simulink model "example_iec61850"  (Simulink 8.1)
settings: Solver=FixedStepDiscrete  SolverMode=SingleTasking  StartTime=0.0  StopTime=Inf  FixedStep=0.00025  RelTol=1e-3
PostLoadFcn:
  | Ts=0.02; Ns=4; txnb=0; rxnb=0;
InitFcn:
  | Ts=0.02; Ns=4; txnb=0; rxnb=0;
undefined symbols (not defined in the file): CD
libraries: opal_lib x6, simulink x6, rtio_iec61850 x4, rtlab x2
settings Model: Creator=CristinaO  LastModifiedBy=pkoralew  BufferReuse=off
settings DataIOCC: SaveOutput=off  SignalLogging=off  SaveTime=off
settings OptimizationCC: BlockReduction=off  OptimizeBlockIOStorage=off  BufferReuse=off  ExpressionFolding=off  LocalBlockOutputs=off  InitFltsAndDblsToZero=on
settings DebuggingCC: SaveWithParameterizedLinksMsg=none  StrictBusMsg=Warning
settings HardwareCC: TargetHWDeviceType=32-bit Generic
settings GRTTargetCC: TargetFcnLib=ansi_tfl_tmw.mat

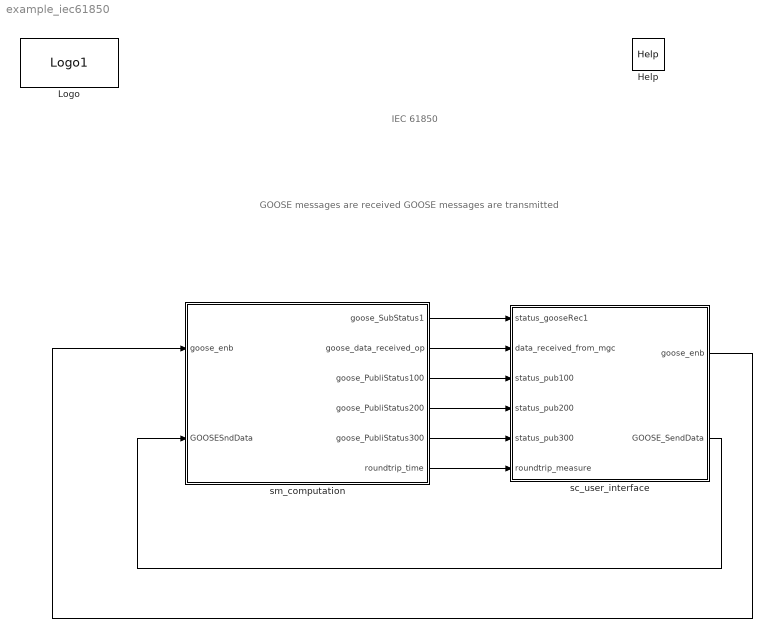
== system example_iec61850 ==
  note: GOOSE messages are received
      |
      | GOOSE messages are transmitted
  note: IEC 61850
  Help : opal_lib/Help  docfile=../help/help.html
  Logo : opal_lib/Logo1  vide=[]
  sc_user_interface : Subsystem
  sm_computation : Subsystem
  wires:
  sm_computation/1(goose_SubStatus1) -> sc_user_interface/1(status_gooseRec1)
  sm_computation/2(goose_data_received_op) -> sc_user_interface/2(data_received_from_mgc)
  sc_user_interface/1(goose_enb) -> sm_computation/1(goose_enb)
  sc_user_interface/2(GOOSE_SendData) -> sm_computation/2(GOOSESndData)
  sm_computation/3("goose_PubliStatus100 ") -> sc_user_interface/3(status_pub100)
  sm_computation/4(goose_PubliStatus200) -> sc_user_interface/4(status_pub200)
  sm_computation/5(goose_PubliStatus300) -> sc_user_interface/5(status_pub300)
  sm_computation/6(roundtrip_time) -> sc_user_interface/6(roundtrip_measure)

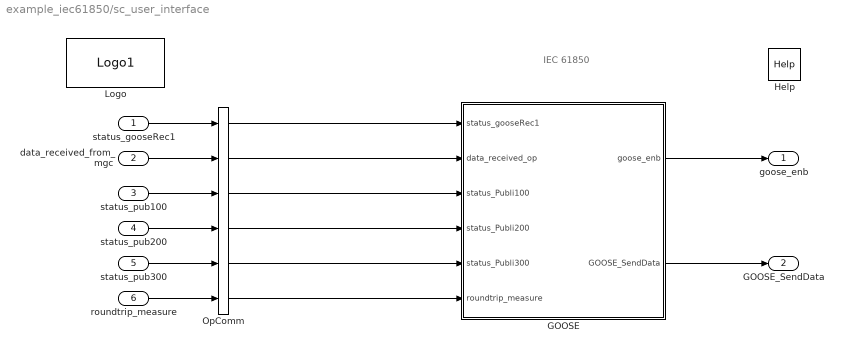
== system example_iec61850/sc_user_interface ==
  note: IEC 61850
  status_gooseRec1 : Inport
  data_received_from_mgc : Inport  Port=2
  status_pub100 : Inport  Port=3
  status_pub200 : Inport  Port=4
  status_pub300 : Inport  Port=5
  roundtrip_measure : Inport  Port=6
  GOOSE : Subsystem
  Help : opal_lib/Help  docfile=../help/help.html
  Logo : opal_lib/Logo1  vide=[]
  OpComm : rtlab/OpComm  nbport=6  groupe_acq=1  subsys_rate=0  st=0  Synchronization=off  Interpolation=off  Threshold=1.0  Missed_Data=off  Sim_Time=off  Samples=off  dynSigOut=off  from_console=0  warning_done=off  writeOpCommFile=off  Offset=off
  goose_enb : Outport
  GOOSE_SendData : Outport  Port=2
  wires:
  status_gooseRec1/1 -> OpComm/1
  data_received_from_mgc/1 -> OpComm/2
  GOOSE/1(goose_enb) -> goose_enb/1
  GOOSE/2(GOOSE_SendData) -> GOOSE_SendData/1
  OpComm/1 -> GOOSE/1(status_gooseRec1)
  OpComm/2 -> GOOSE/2(data_received_op)
  status_pub300/1 -> OpComm/5
  status_pub100/1 -> OpComm/3
  status_pub200/1 -> OpComm/4
  OpComm/5 -> GOOSE/5(status_Publi300)
  OpComm/3 -> GOOSE/3(status_Publi100)
  OpComm/4 -> GOOSE/4(status_Publi200)
  roundtrip_measure/1 -> OpComm/6
  OpComm/6 -> GOOSE/6(roundtrip_measure)

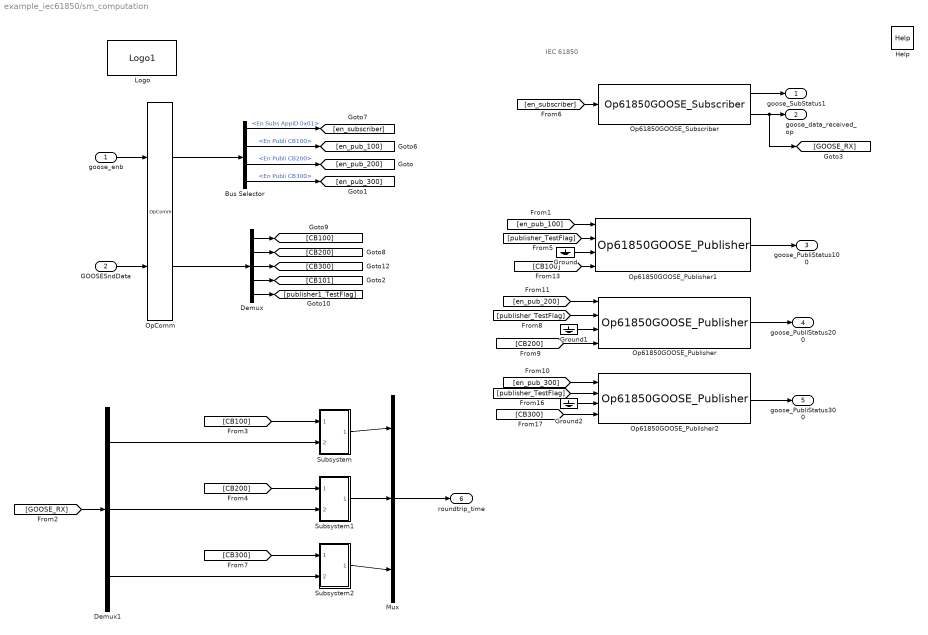
== system example_iec61850/sm_computation ==
  note: IEC 61850
  goose_enb : Inport
  GOOSESndData : Inport  Port=2
  Bus Selector : BusSelector  OutputSignals=En Subs AppID 0x01,En Publi CB100,En Publi CB200,En Publi CB300
  Demux : Demux  Outputs=5
  Demux1 : Demux  Outputs=3
  Ground : Ground
  Ground1 : Ground
  Ground2 : Ground
  Help : opal_lib/Help  docfile=../help/help.html
  Logo : opal_lib/Logo1  vide=[]
  Mux : Mux  Inputs=3
  Op61850GOOSE_Publisher : rtio_iec61850/Op61850GOOSE_Publisher  nic_name=eth1  ied_name=CB200  select_scl=off  scl_file=CB200.icd  scl_fullpath=.  goose_name=Goose_TRIP1  goose_msgid=0x0200  mac_address=01-0C-CD-01-28-50  vlan_prio=4  vlan_id=000  mintime=25  maxtime=250  gocbref=CB200LDevice1/LLN0$GO$CB_Goose_TRIP1  dataset=CB200LDevice1/LLN0$Goose_TRIP1  goID=Goose_TRIP1  confrev=1  externalClock=off
      settings: AttributesFormatString=%<Name>\nAppId = %<goose_msgid>
  Op61850GOOSE_Publisher1 : rtio_iec61850/Op61850GOOSE_Publisher  nic_name=eth1  ied_name=CB100  select_scl=off  scl_file=CB100.icd  scl_fullpath=.  goose_name=Goose_TRIP1  goose_msgid=0x0100  mac_address=01-0C-CD-01-28-50  vlan_prio=4  vlan_id=000  mintime=25  maxtime=250  gocbref=CB100LDevice1/LLN0$GO$CB_Goose_TRIP1  dataset=CB100LDevice1/LLN0$Goose_TRIP1  goID=Goose_TRIP1  confrev=1  externalClock=off
      settings: AttributesFormatString=%<Name>\nAppId = %<goose_msgid>
  Op61850GOOSE_Publisher2 : rtio_iec61850/Op61850GOOSE_Publisher  nic_name=eth1  ied_name=CB300  select_scl=off  scl_file=CB300.icd  scl_fullpath=.  goose_name=Goose_TRIP1  goose_msgid=0x0300  mac_address=01-0C-CD-01-28-50  vlan_prio=4  vlan_id=000  mintime=25  maxtime=250  gocbref=CB300LDevice1/LLN0$GO$CB_Goose_TRIP1  dataset=CB300LDevice1/LLN0$Goose_TRIP1  goID=Goose_TRIP1  confrev=1  externalClock=off
      settings: AttributesFormatString=%<Name>\nAppId = %<goose_msgid>
  Op61850GOOSE_Subscriber : rtio_iec61850/Op61850GOOSE_Subscriber  nic_name=eth1  ied_name=MGC  select_scl=off  scl_file=MGC.icd  scl_fullpath=.  goose_name=Goose_TRIP1  goose_msgid=0x0001  mac_address=01-0C-CD-01-28-60
      settings: AttributesFormatString=%<Name>\nAppId = %<goose_msgid>
  OpComm : rtlab/OpComm  nbport=2  groupe_acq=1  subsys_rate=0  st=0  Synchronization=on  Interpolation=on  Threshold=1.0  Missed_Data=off  Sim_Time=off  Samples=off  dynSigOut=off  from_console=1  warning_done=off  writeOpCommFile=off  Offset=off
  Subsystem : Subsystem
  Subsystem1 : Subsystem
  Subsystem2 : Subsystem
  goose_SubStatus1 : Outport
  goose_data_received_op : Outport  Port=2
  "goose_PubliStatus100 " : Outport  Port=3
  goose_PubliStatus200 : Outport  Port=4
  goose_PubliStatus300 : Outport  Port=5
  roundtrip_time : Outport  Port=6
  wires:
  goose_enb/1 -> OpComm/1
  Op61850GOOSE_Subscriber/1 -> goose_SubStatus1/1
  OpComm/1 -> Bus Selector/1
  GOOSESndData/1 -> OpComm/2
  Bus Selector/1 -> [en_subscriber]  "<En Subs AppID 0x01>"
  Bus Selector/2 -> [en_pub_100]  "<En Publi CB100>"
  Bus Selector/3 -> [en_pub_200]  "<En Publi CB200>"
  Bus Selector/4 -> [en_pub_300]  "<En Publi CB300>"
  [en_subscriber] -> Op61850GOOSE_Subscriber/1
  OpComm/2 -> Demux/1
  Demux/1 -> [CB100]
  Demux/2 -> [CB200]
  Demux/3 -> [CB300]
  Demux/4 -> [CB101]
  Demux/5 -> [publisher1_TestFlag]
  [publisher_TestFlag] -> Op61850GOOSE_Publisher/2
  [publisher_TestFlag] -> Op61850GOOSE_Publisher1/2
  Op61850GOOSE_Publisher1/1 -> "goose_PubliStatus100 "/1
  [en_pub_200] -> Op61850GOOSE_Publisher/1
  [en_pub_100] -> Op61850GOOSE_Publisher1/1
  [CB200] -> Op61850GOOSE_Publisher/4
  [CB100] -> Op61850GOOSE_Publisher1/4
  Op61850GOOSE_Publisher/1 -> goose_PubliStatus200/1
  Ground1/1 -> Op61850GOOSE_Publisher/3
  Ground/1 -> Op61850GOOSE_Publisher1/3
  [publisher_TestFlag] -> Op61850GOOSE_Publisher2/2
  [en_pub_300] -> Op61850GOOSE_Publisher2/1
  [CB300] -> Op61850GOOSE_Publisher2/4
  Op61850GOOSE_Publisher2/1 -> goose_PubliStatus300/1
  Ground2/1 -> Op61850GOOSE_Publisher2/3
  Op61850GOOSE_Subscriber/2 -> goose_data_received_op/1, [GOOSE_RX]
  [GOOSE_RX] -> Demux1/1
  [CB100] -> Subsystem/1(In1)
  Demux1/1 -> Subsystem/2(In2)
  Subsystem/1(Out1) -> Mux/1
  [CB200] -> Subsystem1/1(In1)
  Demux1/2 -> Subsystem1/2(In2)
  Subsystem1/1(Out1) -> Mux/2
  [CB300] -> Subsystem2/1(In1)
  Demux1/3 -> Subsystem2/2(In2)
  Subsystem2/1(Out1) -> Mux/3
  Mux/1 -> roundtrip_time/1

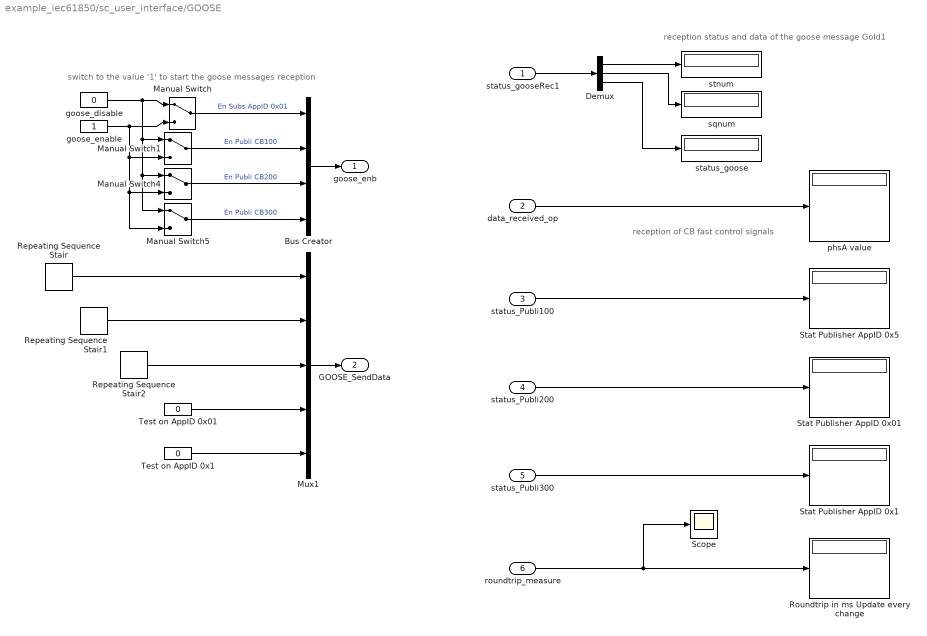
== system example_iec61850/sc_user_interface/GOOSE ==
  note: switch to the value '1' to start the goose messages reception
  note: reception status and data of the goose message GoId1
  note: reception of CB fast control signals
  status_gooseRec1 : Inport
  data_received_op : Inport  Port=2
  status_Publi100 : Inport  Port=3
  status_Publi200 : Inport  Port=4
  status_Publi300 : Inport  Port=5
  roundtrip_measure : Inport  Port=6
  Bus Creator : BusCreator
  Demux : Demux  Outputs=3
  Manual Switch{,1,4..5} (4 alike) : ManualSwitch
  Mux1 : Mux  Inputs=5
  Repeating Sequence Stair : simulink/Sources/Repeating Sequence Stair  OutValues=[0 1 0 1 0 1 0 1].'  tsamp=3  OutMin=[]  OutMax=[]  OutDataTypeStr=double  OutputDataTypeScalingMode=double  OutDataType=fixdt(0,8)  ConRadixGroup=Best Precision: Vector-wise  OutScaling=2^-12
  Repeating Sequence Stair1 : simulink/Sources/Repeating Sequence Stair  OutValues=[0 1 0 1 0 1 0 1].'  tsamp=2.900250  OutMin=[]  OutMax=[]  OutDataTypeStr=double  OutputDataTypeScalingMode=double  OutDataType=fixdt(0,8)  ConRadixGroup=Best Precision: Vector-wise  OutScaling=2^-12
  Repeating Sequence Stair2 : simulink/Sources/Repeating Sequence Stair  OutValues=[0 1 0 1 0 1 0 1].'  tsamp=2.800250  OutMin=[]  OutMax=[]  OutDataTypeStr=double  OutputDataTypeScalingMode=double  OutDataType=fixdt(0,8)  ConRadixGroup=Best Precision: Vector-wise  OutScaling=2^-12
  Roundtrip in ms Update every change : Display
  Scope : Scope
      settings: Decimation=100
  Stat Publisher AppID 0x01 : Display
  Stat Publisher AppID 0x1 : Display
  Stat Publisher AppID 0x5 : Display
  Test on AppID 0x01 : Constant  Value=0
  Test on AppID 0x1 : Constant  Value=0
  goose_disable : Constant  Value=0
  goose_enable : Constant
  phsA value : Display
  sqnum : Display
  status_goose : Display
  stnum : Display
  goose_enb : Outport
  GOOSE_SendData : Outport  Port=2
  wires:
  goose_disable/1 -> Manual Switch/1, Manual Switch1/1, Manual Switch4/1, Manual Switch5/1
  goose_enable/1 -> Manual Switch/2, Manual Switch1/2, Manual Switch4/2, Manual Switch5/2
  Repeating Sequence Stair/1 -> Mux1/1
  Repeating Sequence Stair1/1 -> Mux1/2
  Mux1/1 -> GOOSE_SendData/1
  Repeating Sequence Stair2/1 -> Mux1/3
  Test on AppID 0x01/1 -> Mux1/4
  Bus Creator/1 -> goose_enb/1
  Manual Switch/1 -> Bus Creator/1  "En Subs AppID 0x01"
  Manual Switch1/1 -> Bus Creator/2  "En Publi CB100"
  Manual Switch4/1 -> Bus Creator/3  "En Publi CB200"
  Manual Switch5/1 -> Bus Creator/4  "En Publi CB300"
  status_gooseRec1/1 -> Demux/1
  status_Publi100/1 -> Stat Publisher AppID 0x5/1
  status_Publi200/1 -> Stat Publisher AppID 0x01/1
  Demux/3 -> status_goose/1
  data_received_op/1 -> phsA value/1
  Demux/1 -> stnum/1
  Demux/2 -> sqnum/1
  Test on AppID 0x1/1 -> Mux1/5
  status_Publi300/1 -> Stat Publisher AppID 0x1/1
  roundtrip_measure/1 -> Scope/1, Roundtrip in ms Update every change/1

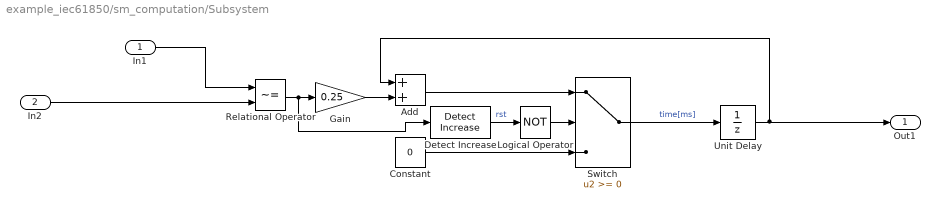
== system example_iec61850/sm_computation/Subsystem ==
  In1 : Inport
  In2 : Inport  Port=2
  Add : Sum
  Constant : Constant  Value=0
  Detect Increase : simulink/Logic and Bit Operations/Detect Increase  vinit=0.0  InputProcessing=Inherited  OutDataTypeStr=boolean
  Gain : Gain  Gain=0.25
  Logical Operator : Logic  Operator=NOT  AllPortsSameDT=off  OutDataTypeStr=boolean
  Relational Operator : RelationalOperator  Operator=~=  OutDataTypeStr=boolean
  Switch : Switch
  Unit Delay : UnitDelay  SampleTime=-1
  Out1 : Outport
  wires:
  Relational Operator/1 -> Detect Increase/1, Gain/1
  In1/1 -> Relational Operator/1
  Logical Operator/1 -> Switch/2
  Gain/1 -> Add/2
  Add/1 -> Switch/1
  Unit Delay/1 -> Out1/1, Add/1
  In2/1 -> Relational Operator/2
  Switch/1 -> Unit Delay/1  "time[ms]"
  Constant/1 -> Switch/3
  Detect Increase/1 -> Logical Operator/1  "rst"

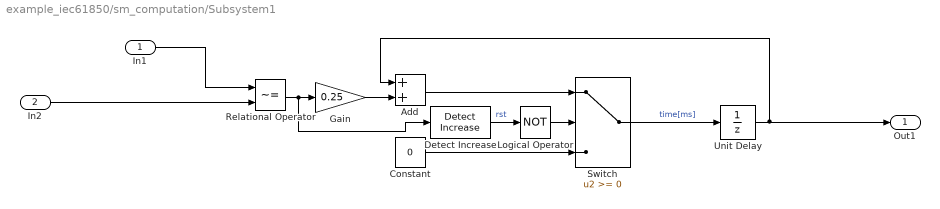
== system example_iec61850/sm_computation/Subsystem1 ==
  In1 : Inport
  In2 : Inport  Port=2
  Add : Sum
  Constant : Constant  Value=0
  Detect Increase : simulink/Logic and Bit Operations/Detect Increase  vinit=0.0  InputProcessing=Inherited  OutDataTypeStr=boolean
  Gain : Gain  Gain=0.25
  Logical Operator : Logic  Operator=NOT  AllPortsSameDT=off  OutDataTypeStr=boolean
  Relational Operator : RelationalOperator  Operator=~=  OutDataTypeStr=boolean
  Switch : Switch
  Unit Delay : UnitDelay  SampleTime=-1
  Out1 : Outport
  wires:
  Detect Increase/1 -> Logical Operator/1  "rst"
  Constant/1 -> Switch/3
  Switch/1 -> Unit Delay/1  "time[ms]"
  In2/1 -> Relational Operator/2
  Unit Delay/1 -> Add/1, Out1/1
  Add/1 -> Switch/1
  Gain/1 -> Add/2
  Logical Operator/1 -> Switch/2
  In1/1 -> Relational Operator/1
  Relational Operator/1 -> Gain/1, Detect Increase/1

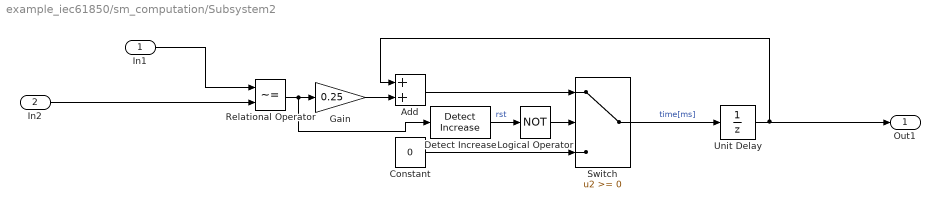
== system example_iec61850/sm_computation/Subsystem2 ==
  In1 : Inport
  In2 : Inport  Port=2
  Add : Sum
  Constant : Constant  Value=0
  Detect Increase : simulink/Logic and Bit Operations/Detect Increase  vinit=0.0  InputProcessing=Inherited  OutDataTypeStr=boolean
  Gain : Gain  Gain=0.25
  Logical Operator : Logic  Operator=NOT  AllPortsSameDT=off  OutDataTypeStr=boolean
  Relational Operator : RelationalOperator  Operator=~=  OutDataTypeStr=boolean
  Switch : Switch
  Unit Delay : UnitDelay  SampleTime=-1
  Out1 : Outport
  wires:
  Relational Operator/1 -> Detect Increase/1, Gain/1
  In1/1 -> Relational Operator/1
  Logical Operator/1 -> Switch/2
  Gain/1 -> Add/2
  Add/1 -> Switch/1
  Unit Delay/1 -> Out1/1, Add/1
  In2/1 -> Relational Operator/2
  Switch/1 -> Unit Delay/1  "time[ms]"
  Constant/1 -> Switch/3
  Detect Increase/1 -> Logical Operator/1  "rst"
